simulink model "SequencingTest"  (R2018b)
settings: Solver=VariableStepAuto  StartTime=0.0  StopTime=100  RelTol=1e-3
undefined symbols (not defined in the file or in its folder): m, n
settings Model: Creator=tas5  LastModifiedBy=tas5

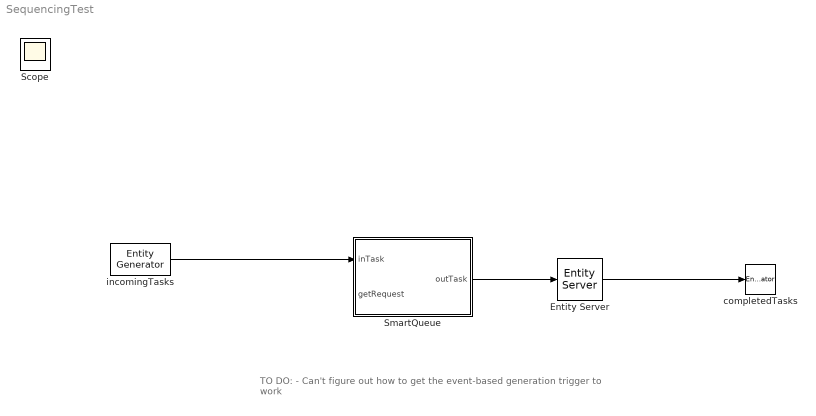
== system SequencingTest ==
  note: TO DO:
      | - Can't figure out how to get the event-based generation trigger to work
  Entity Server : EntityServer  InputPortMessageModes=m  OutputPortMessageModes=m  Capacity=1
  SmartQueue : Subsystem  InitFcn=|
      | coder.extrinsic('evalin')
      | 
      | productInstances = [];
      | productIDs = [];
      | availableTasks = [];
      | completedTasks = [];
      | 
      | evalin('base', 'QueueController = Controller;')
      | evalin('base', 'sq1 = RandomSequencing;')
      | evalin('base','QueueController.Sequencing = sq1;');
  completedTasks : EntityTerminator  InputPortMessageModes=m  EntryAction=|
      | coder.extrinsic('evalin');
      | coder.extrinsic('assignin');
      | coder.extrinsic('num2str');
      | coder.extrinsic('strcat')
      | coder.extrinsic('now');
      | 
      | %Read the queue list from workspace, then write new entity to it
      | %Return to workspace
      | simTime = evalin('base', 'get_param(''SequencingTest'',''SimulationTime'');');
      | completedTasks = evalin('base', 'completedTasks');
      | completedTasks = [completedTasks; [simTime, entity.serialNumber, entity.productTypeID, entity.color]];
      | assignin('base', 'completedTasks', completedTasks);
      | 
      | evalin('base', strcat('part = productInstances{[productIDs == ', num2str(entity.serialNumber), ']};', ...
      |     'part.actualCompleteTime = ', num2str(simTime), ';', ...
      |     'part.processPlan.actualCompleteTime = ', num2str(simTime), ';'));
  incomingTasks : EntityGenerator  OutputPortMessageModes=m  GenerateAction=|  ExitAction=|  AttributeName=serialNumber|productTypeID|color|nextNode|serviceTime|priority  AttributeInitialValue=1|1|1|5|1|0  EntityType=Structured  EntityTypeName=Task
      GenerateAction=|
      | coder.extrinsic('randi');
      | persistent idx;
      | persistent rngInit;
      | if isempty(idx)
      |     idx = 1;
      | end
      | if isempty(rngInit)
      |     seed = 12345;
      |     rng(seed);
      |     rngInit = true;
      | end
      | 
      | entity.serialNumber = idx;
      | entity.productTypeID = randi(2,1); %randi(5,1);
      | entity.color = randi(3,1);
      | 
      | idx = idx + 1;
      ExitAction=|
      | coder.extrinsic('evalin')
      | coder.extrinsic('strcat')
      | coder.extrinsic('num2str')
      | 
      | productTypeIDTable = {'ProductX001', 'ProductY001'};
      | 
      | productTypeID = productTypeIDTable{entity.productTypeID};
      | evalin('base', strcat('productInstances{end+1} = ', productTypeID, '(', num2str(entity.serialNumber), ');'))
      | evalin('base', strcat('productIDs(end+1) = ', num2str(entity.serialNumber), ';'));
      | 
      | 
      | evalin('base', strcat('part = productInstances{[productIDs == ', num2str(entity.serialNumber), ']};', ...
      |     'QueueController.createProductListener(part);', ...    
      |     'part.processPlan.actualStartTime = get_param(''SequencingTest'',''SimulationTime'');'));
  Scope : Scope
  wires:
  incomingTasks/1 -> SmartQueue/1(inTask)
  SmartQueue/1(outTask) -> Entity Server/1
  Entity Server/1 -> completedTasks/1

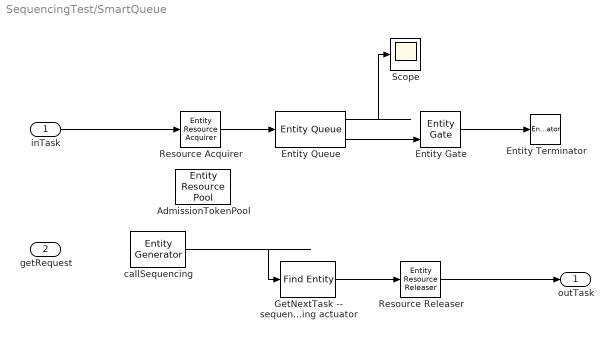
== system SequencingTest/SmartQueue ==
  inTask : Inport
  getRequest : Inport  Port=2
  AdmissionTokenPool : EntityResourcePool  ResourceName=AdmissionToken  ResourceAmount=100
  Entity Gate : EntityGate  InputPortMessageModes=m,m  OutputPortMessageModes=m
  Entity Queue : EntityQueue  InputPortMessageModes=m  OutputPortMessageModes=n,m  EntryAction=|  AverageWait=on
      | coder.extrinsic('evalin');
      | coder.extrinsic('assignin');
      | coder.extrinsic('now');
      | 
      | %Read the queue list from workspace, then write new entity to it
      | %Return to workspace
      | availableTasks = evalin('base', 'availableTasks');
      | availableTasks = [availableTasks; [0, now, entity.serialNumber, entity.productTypeID, entity.color]];
      | assignin('base', 'availableTasks', availableTasks);
      settings: OutputPortMap=o2,o5
  Entity Terminator : EntityTerminator  InputPortMessageModes=m
  "GetNextTask -- sequencing actuator" : FindEntity  InputPortMessageModes=m  OutputPortMessageModes=m  ResourceName=AdmissionToken  EnableOutput=on  EntityFilter=on  MatchingCondition=|  NumberEntitiesFound=on
      | %coder.extrinsic('evalin')
      | %index = evalin('base', 'Sequencing(availableTasks);')
      | %match = isequal(index, entity.ID);
      | 
      | match = isequal(trigger.selectedID, entity.serialNumber);
      settings: OutputPortMap=o6
  Resource Acquirer : EntityResourceAcquirer  InputPortMessageModes=m  OutputPortMessageModes=m  NumberWaitingEntities=100  ResourceName=AdmissionToken
      settings: OutputPortMap=o3
  Resource Releaser : EntityResourceReleaser  InputPortMessageModes=m  OutputPortMessageModes=m  ResourceToRelease=Selected  ResourceName=AdmissionToken
  Scope : Scope
  callSequencing : EntityGenerator  OutputPortMessageModes=m  Period=2  GenerateEntityAtSimulationStart=off  GenerateAction=|  AttributeName=selectedID  EntityType=Structured  EntityTypeName=trigger  EntityPriority=100
      | coder.extrinsic('evalin')
      | %coder.extrinsic('assignin')
      | %coder.extrinsic('sortrows')
      | %coder.extrinsic('min')
      | %coder.extrinsic('Sequencing')
      | 
      | entity.selectedID = evalin('base', 'QueueController.Sequencing.Sequencing(availableTasks);')
      | 
      | 
      | %queuedEntity = evalin('base', 'queuedEntity');
      | %call sequencing
      | %[B,I] = sortrows(queuedEntity, [4,5,2]);
      | %queuedEntity(:,1) = I;
      | %[Y, J] = min(I);
      | %assignin('base','queuedEntity', B);
      | %evalin('base', 'queuedEntity(1,:) = []');
      | %entity.selectedID = queuedEntity(J,3);
  outTask : Outport
  wires:
  callSequencing/1 -> "GetNextTask -- sequencing actuator"/1
  inTask/1 -> Resource Acquirer/1
  "GetNextTask -- sequencing actuator"/1 -> Resource Releaser/1
  Resource Releaser/1 -> outTask/1
  Entity Queue/2 -> Entity Gate/2
  Entity Gate/1 -> Entity Terminator/1
  Resource Acquirer/1 -> Entity Queue/1
  Entity Queue/1 -> Scope/1
